simulink model "FlatEarth_MATLAB6"  (Simulink 4.00)
settings: Solver=ode45  StartTime=0.0  StopTime=10.0  RelTol=1e-3
undefined symbols (not defined in the file or in its folder): constant, uIC, xIC
settings Model: LastModifiedBy=andrisan

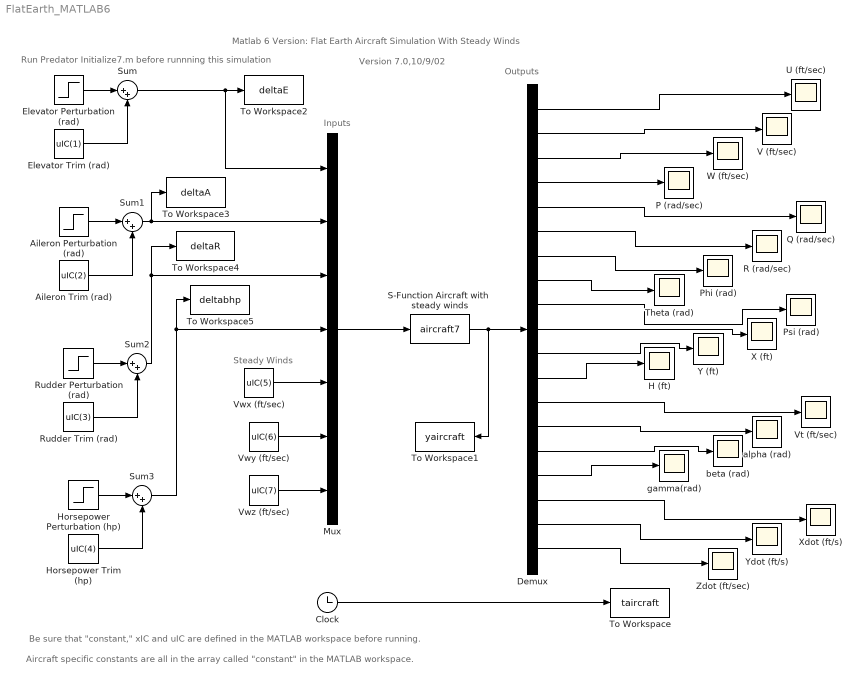
== system FlatEarth_MATLAB6 ==
  note: Matlab 6 Version: Flat Earth Aircraft Simulation With Steady Winds
  note: Version 7.0,10/9/02
  note: Be sure that "constant," xIC and uIC are defined in the MATLAB workspace before running.
  note: Aircraft specific constants are all in the array called "constant" in the MATLAB workspace.
  note: Steady Winds
  note: Inputs
  note: Outputs
  note: Run Predator Initialize7.m before runnning this simulation
  Aileron Perturbation (rad) : Step  Time=1  Before=0  After=0  SampleTime=0
  Aileron Trim (rad) : Constant  Value=uIC(2)
  Clock : Clock
      settings: DisplayTime=off  Decimation=10
  Demux : Demux  Outputs=19  BusSelectionMode=off
  Elevator Perturbation (rad) : Step  Time=1  Before=0  After=0  SampleTime=0
  Elevator Trim (rad) : Constant  Value=uIC(1)
  H (ft) : Scope
      settings: TimeRange=auto  YMin=-5  YMax=5  SaveToWorkspace=off  SaveName=ScopeData11  LimitDataPoints=on  MaxDataPoints=5000
  Horsepower Perturbation (hp) : Step  Time=1  Before=0  After=0  SampleTime=0
  Horsepower Trim (hp) : Constant  Value=uIC(4)
  Mux : Mux  Inputs=7
  P (rad/sec) : Scope
      settings: TimeRange=auto  YMin=-5  YMax=5  SaveToWorkspace=off  SaveName=ScopeData3  LimitDataPoints=on  MaxDataPoints=5000
  Phi (rad) : Scope
      settings: TimeRange=auto  YMin=-5  YMax=5  SaveToWorkspace=off  SaveName=ScopeData6  LimitDataPoints=on  MaxDataPoints=5000
  Psi (rad) : Scope
      settings: TimeRange=auto  YMin=-5  YMax=5  SaveToWorkspace=off  SaveName=ScopeData8  LimitDataPoints=on  MaxDataPoints=5000
  Q (rad/sec) : Scope
      settings: TimeRange=auto  YMin=-5  YMax=5  SaveToWorkspace=off  SaveName=ScopeData4  LimitDataPoints=on  MaxDataPoints=5000
  R (rad/sec) : Scope
      settings: TimeRange=auto  YMin=-5  YMax=5  SaveToWorkspace=off  SaveName=ScopeData5  LimitDataPoints=on  MaxDataPoints=5000
  Rudder Perturbation (rad) : Step  Time=1  Before=0  After=-10/57.3  SampleTime=0
  Rudder Trim (rad) : Constant  Value=uIC(3)
  S-Function Aircraft with  steady winds : S-Function  FunctionName=aircraft7  Parameters=constant,xIC  PortCounts=[]  SFunctionModules=''
  Sum{,1..3} (4 alike) : Sum  Inputs=|++  SaturateOnIntegerOverflow=on
  Theta (rad) : Scope
      settings: TimeRange=auto  YMin=-5  YMax=5  SaveToWorkspace=off  SaveName=ScopeData7  LimitDataPoints=on  MaxDataPoints=5000
  To Workspace : ToWorkspace  VariableName=taircraft  SampleTime=-1  SaveFormat=Array
  To Workspace1 : ToWorkspace  VariableName=yaircraft  SampleTime=-1  SaveFormat=Array
  To Workspace2 : ToWorkspace  VariableName=deltaE  SampleTime=-1  SaveFormat=Array
  To Workspace3 : ToWorkspace  VariableName=deltaA  SampleTime=-1  SaveFormat=Array
  To Workspace4 : ToWorkspace  VariableName=deltaR  SampleTime=-1  SaveFormat=Array
  To Workspace5 : ToWorkspace  VariableName=deltabhp  SampleTime=-1  SaveFormat=Array
  U (ft/sec) : Scope
      settings: TimeRange=auto  YMin=-5  YMax=5  SaveToWorkspace=off  SaveName=ScopeData  LimitDataPoints=on  MaxDataPoints=5000
  V (ft/sec) : Scope
      settings: TimeRange=auto  YMin=-5  YMax=5  SaveToWorkspace=off  LimitDataPoints=on  MaxDataPoints=5000
  Vt (ft/sec) : Scope
      settings: TimeRange=auto  YMin=-5  YMax=5  SaveToWorkspace=off  SaveName=ScopeData12  LimitDataPoints=on  MaxDataPoints=5000
  Vwx (ft/sec) : Constant  Value=uIC(5)
  Vwy (ft/sec) : Constant  Value=uIC(6)
  Vwz (ft/sec) : Constant  Value=uIC(7)
  W (ft/sec) : Scope
      settings: TimeRange=auto  YMin=0  YMax=14  SaveToWorkspace=off  SaveName=ScopeData2  LimitDataPoints=on  MaxDataPoints=5000
  X (ft) : Scope
      settings: TimeRange=auto  YMin=-5  YMax=5  SaveToWorkspace=off  SaveName=ScopeData9  LimitDataPoints=on  MaxDataPoints=5000
  Xdot (ft/s) : Scope
      settings: TimeRange=auto  YMin=-5  YMax=5  SaveToWorkspace=off  SaveName=ScopeData16  LimitDataPoints=on  MaxDataPoints=5000
  Y (ft) : Scope
      settings: TimeRange=auto  YMin=-5  YMax=5  SaveToWorkspace=off  SaveName=ScopeData10  LimitDataPoints=on  MaxDataPoints=5000
  Ydot (ft/s) : Scope
      settings: TimeRange=auto  YMin=-5  YMax=5  SaveToWorkspace=off  SaveName=ScopeData17  LimitDataPoints=on  MaxDataPoints=5000
  Zdot (ft/sec) : Scope
      settings: TimeRange=auto  YMin=-5  YMax=5  SaveToWorkspace=off  SaveName=ScopeData18  LimitDataPoints=on  MaxDataPoints=5000
  alpha (rad) : Scope
      settings: TimeRange=auto  YMin=-5  YMax=5  SaveToWorkspace=off  SaveName=ScopeData13  LimitDataPoints=on  MaxDataPoints=5000
  beta (rad) : Scope
      settings: TimeRange=auto  YMin=-5  YMax=5  SaveToWorkspace=off  SaveName=ScopeData14  LimitDataPoints=on  MaxDataPoints=5000
  gamma(rad) : Scope
      settings: TimeRange=auto  YMin=-5  YMax=5  SaveToWorkspace=off  SaveName=ScopeData15  LimitDataPoints=on  MaxDataPoints=5000
  wires:
  Demux/1 -> U (ft/sec)/1
  Demux/2 -> V (ft/sec)/1
  Demux/3 -> W (ft/sec)/1
  Demux/4 -> P (rad/sec)/1
  Demux/5 -> Q (rad/sec)/1
  Demux/6 -> R (rad/sec)/1
  Demux/7 -> Phi (rad)/1
  Demux/8 -> Theta (rad)/1
  Demux/9 -> Psi (rad)/1
  Demux/10 -> X (ft)/1
  Demux/11 -> Y (ft)/1
  Demux/12 -> H (ft)/1
  Demux/13 -> Vt (ft/sec)/1
  Demux/14 -> alpha (rad)/1
  Demux/15 -> beta (rad)/1
  Demux/16 -> gamma(rad)/1
  Demux/17 -> Xdot (ft/s)/1
  Demux/18 -> Ydot (ft/s)/1
  Demux/19 -> Zdot (ft/sec)/1
  Clock/1 -> To Workspace/1
  S-Function Aircraft with  steady winds/1 -> Demux/1, To Workspace1/1
  Elevator Perturbation (rad)/1 -> Sum/1
  Elevator Trim (rad)/1 -> Sum/2
  Aileron Perturbation (rad)/1 -> Sum1/1
  Aileron Trim (rad)/1 -> Sum1/2
  Rudder Perturbation (rad)/1 -> Sum2/1
  Rudder Trim (rad)/1 -> Sum2/2
  Horsepower Perturbation (hp)/1 -> Sum3/1
  Horsepower Trim (hp)/1 -> Sum3/2
  Sum/1 -> Mux/1, To Workspace2/1
  Sum1/1 -> Mux/2, To Workspace3/1
  Sum2/1 -> Mux/3, To Workspace4/1
  Sum3/1 -> Mux/4, To Workspace5/1
  Vwx (ft/sec)/1 -> Mux/5
  Vwy (ft/sec)/1 -> Mux/6
  Vwz (ft/sec)/1 -> Mux/7
  Mux/1 -> S-Function Aircraft with  steady winds/1
